simulink model "AIE_RTL_cosim_black_box"  (R2019b)
settings: Solver=VariableStepAuto  StartTime=0.0  StopTime=4000  RelTol=1e-3
InitFcn:
  | xmcCheckSlxPath(bdroot);
  | input = readcomplexdata('./sw/input.h');
  | 
  | % ii of the SysGen black box design is 19. Hence we are running
  | % the sysgen desgin at 20 times faster than
  | % the input sample time.
  | 
  | sample_time = 0.5/20
undefined symbols (not defined in the file or in its folder): c, xc7vx485tffg1157
libraries: xbsIndex_r4 x5, ModelComposer x5, dspsrcs4 x1
settings Model: Creator=abehbood  LastModifiedBy=abehbood
settings SFSimCC: CustomCodeUndefinedFunction=UseInterfaceOnly

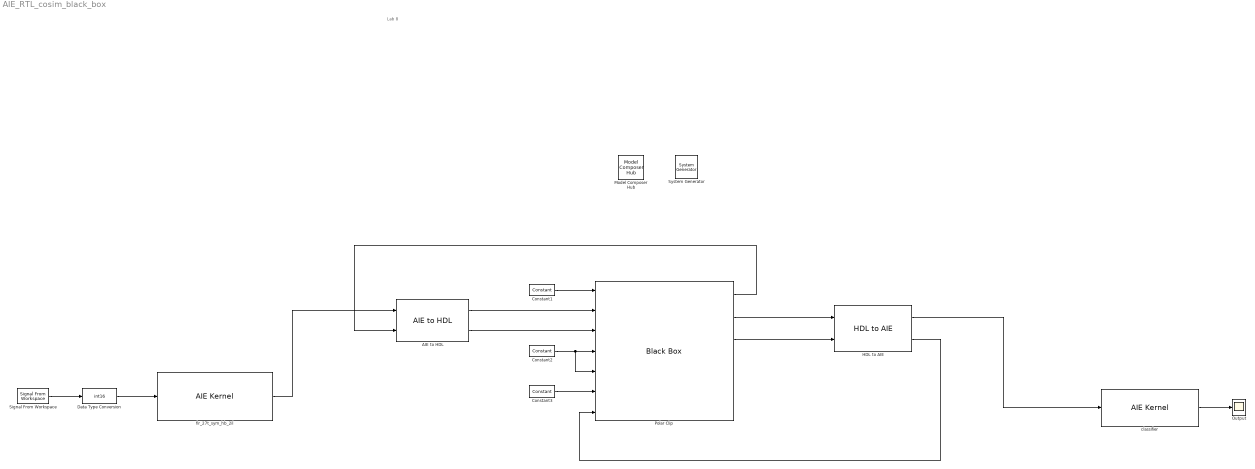
== system AIE_RTL_cosim_black_box ==
  note: Lab 8
  " System Generator" : xbsIndex_r4/ System Generator  Tag=genX  xilinxfamily=kintex7  part=xc7k325t  speed=-3  package=fbg676  synthesis_tool=Vivado  clock_wrapper=Clock Enables  directory=./netlist  proj_type=Vivado  Synth_file=Vivado Synthesis Defaults  Impl_file=Vivado Implementation Defaults  testbench=off  simulink_period=sample_time  sysclk_period=10  dcm_input_clock_period=10  incr_netlist=off  trim_vbits=Everywhere in SubSystem  dbl_ovrd=According to Block Masks  core_generation=According to Block Masks  run_coregen=off  deprecated_control=off  eval_field=0  block_type=sysgen
  AIE to HDL : ModelComposer/AIE to HDL  OutDataType=uint32  OutSampleTime=sample_time
  Constant1 : xbsIndex_r4/Constant  const=1  gui_display_data_type=Boolean  arith_type=Boolean  n_bits=16  bin_pt=14  preci_type=Single  exp_width=8  frac_width=24  explicit_period=on  period=sample_time  equ=P=C  opselect=C  inp2=PCIN>>17  opr=+  inp1=P  carry=CIN  dbl_ovrd=off  block_type=constant
  Constant2 : xbsIndex_r4/Constant  const=15  gui_display_data_type=Fixed-point  arith_type=Unsigned  n_bits=4  bin_pt=0  preci_type=Single  exp_width=8  frac_width=24  explicit_period=on  period=sample_time  equ=P=C  opselect=C  inp2=PCIN>>17  opr=+  inp1=P  carry=CIN  dbl_ovrd=off  block_type=constant
  Constant3 : xbsIndex_r4/Constant  const=0  gui_display_data_type=Boolean  arith_type=Boolean  n_bits=16  bin_pt=14  preci_type=Single  exp_width=8  frac_width=24  explicit_period=on  period=sample_time  equ=P=C  opselect=C  inp2=PCIN>>17  opr=+  inp1=P  carry=CIN  dbl_ovrd=off  block_type=constant
  Data Type Conversion : DataTypeConversion  OutDataTypeStr=int16
  HDL to AIE : ModelComposer/HDL to AIE  OutDataType=int16 (c)  OutSampleTime=.5  SamplesPerFrame=256  TreadySampleTime=sample_time
  Model Composer Hub : ModelComposer/Model Composer Hub  CodeGeneration=off  SubsystemName=AI Engine  TargetDirectory=./code  ExportType=AI Engines  IpVendor=xilinx.com  IpLibrary=hls  IpVersion=1.0  IpHWLanguage=Verilog  AieCompilerOptions={}  CreateTestbench=on  TestbenchStackSize=10  RunAieSim=on  AieSimTimeout=150000  LaunchVitisAnalyzer=off  RunX86Sim=on  X86SimTimeout=10  ProjDevice=xc7vx485tffg1157-1  ProjDevicePart=xc7vx485tffg1157-1  SamplePeriod=-1  ClockFrequency=200  DataPathParallelism=1
  Output : Scope
  Polar Clip : xbsIndex_r4/Black Box  init_code=polar_clip_config  sim_method=ISE Simulator  verbose=off  block_type=blackbox2
  Signal From Workspace : dspsrcs4/Signal From Workspace  X=input  Ts=1  nsamps=128  OutputAfterFinalValue=Setting to zero  ignoreOrWarnInputAndFrameLengths=off  OutputFrames=off
  classifier : ModelComposer/AIE Kernel  PortAttributesTable={ 'Input', 'input', 'input_stream_cint16 *', '', '', '', '';'Output','output','output_window_int32 *','256','','auto','' }  PortAttributesEnablement={'off', 'off', 'off', 'off', 'off', 'off', 'off';'off', 'off', 'off', 'on', 'off', 'on', 'off'}  FormalArgDecls={'input_stream_cint16 * input', 'output_window_int32 * output'}  PortWindowSizes={0.000000000000000000e+00; 2.560000000000000000e+02}  PortWindowMargins={0.000000000000000000e+00; 0.000000000000000000e+00}  PortSynchronicities={'auto'; 'auto'}  PortSignalSizes={0.000000000000000000e+00; 0.000000000000000000e+00}  SimLibPath=''  FunctionTabVisible=on  FunctionDescription=void classifier(input_stream_cint16 * input, output_window_int32 * output)  KernelHeaderFile=src/kernels.h  KernelFunction=classifier  KernelFunctionSelect=<empty>  KernelSourceFile=src/kernels/classifiers/classify.cc  KernelSearchPaths={}  PreProcOptions={}  CoreRuntimeRatio=0.9  KernelLocSpec=off  ColRowLocation=[0 0]
  fir_27t_sym_hb_2il : ModelComposer/AIE Kernel  PortAttributesTable={ 'Input','inputcb','input_window_cint16 *','128','16','auto','';'Output','outputcb','output_window_cint16 *','256','','auto','' }  PortAttributesEnablement={'off', 'off', 'off', 'on', 'on', 'on', 'off';'off', 'off', 'off', 'on', 'off', 'on', 'off'}  FormalArgDecls={'input_window_cint16 * inputcb', 'output_window_cint16 * outputcb'}  PortWindowSizes={1.280000000000000000e+02; 2.560000000000000000e+02}  PortWindowMargins={1.600000000000000000e+01; 0.000000000000000000e+00}  PortSynchronicities={'auto'; 'auto'}  PortSignalSizes={0.000000000000000000e+00; 0.000000000000000000e+00}  SimLibPath=''  FunctionTabVisible=on  FunctionDescription=void fir_27t_sym_hb_2i(input_window_cint16 * inputcb, output_window_cint16 * outputcb)  KernelHeaderFile=src/kernels.h  KernelFunction=fir_27t_sym_hb_2i  KernelFunctionSelect=<empty>  KernelSourceFile=src/kernels/interpolators/hb27_2i.cc  KernelSearchPaths={}  PreProcOptions={}  CoreRuntimeRatio=0.9  KernelLocSpec=off  ColRowLocation=[0 0]
  wires:
  classifier/1 -> Output/1
  HDL to AIE/1 -> classifier/1
  Data Type Conversion/1 -> fir_27t_sym_hb_2il/1
  Signal From Workspace/1 -> Data Type Conversion/1
  fir_27t_sym_hb_2il/1 -> AIE to HDL/1
  Polar Clip/2 -> HDL to AIE/1
  Constant2/1 -> Polar Clip/5, Polar Clip/4
  AIE to HDL/1 -> Polar Clip/2
  Constant1/1 -> Polar Clip/1
  AIE to HDL/2 -> Polar Clip/3
  HDL to AIE/2 -> Polar Clip/7
  Constant3/1 -> Polar Clip/6
  Polar Clip/1 -> AIE to HDL/2
  Polar Clip/3 -> HDL to AIE/2
